simulink model "servo1"  (Simulink 8.1)
settings: Solver=ode45  StartTime=0.0  StopTime=10.0  RelTol=1e-3
undefined symbols (not defined in the file or in its folder): Kv
settings Model: Creator=mainster  LastModifiedBy=mainster
settings OptimizationCC: BlockReduction=off  BooleanDataType=off
settings DebuggingCC: SaveWithParameterizedLinksMsg=none  SignalResolutionControl=TryResolveAllWithWarning  SolverPrmCheckMsg=none  MultiTaskDSMMsg=warning  MultiTaskCondExecSysMsg=none  StrictBusMsg=None
settings HardwareCC: TargetUnknown=on
settings RTWCC: IncludeERTFirstTime=on

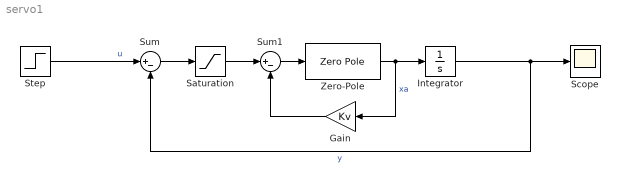
== system servo1 ==
  Gain : Gain  Gain=Kv  SaturateOnIntegerOverflow=on  OutDataTypeStr=Inherit: Same as input  ParamDataTypeStr=Inherit: Same as input
  Integrator : Integrator  InitialCondition=3
  Saturation : Saturate
  Scope : Scope
  Step : Step  Time=0  SampleTime=0
  Sum : Sum  Inputs=|+-  SaturateOnIntegerOverflow=on  InputSameDT=on  OutDataTypeStr=Inherit: Same as first input
  Sum1 : Sum  Inputs=|+-  SaturateOnIntegerOverflow=on  InputSameDT=on  OutDataTypeStr=Inherit: Same as first input
  Zero-Pole : ZeroPole  Zeros=[ ]  Poles=[-5 -1]  Gain=[5]
  wires:
  Sum/1 -> Saturation/1
  Sum1/1 -> Zero-Pole/1
  Zero-Pole/1 -> Integrator/1, Gain/1  "xa"
  Gain/1 -> Sum1/2
  Saturation/1 -> Sum1/1
  Step/1 -> Sum/1  "u"
  Integrator/1 -> Scope/1, Sum/2  "y"
